simulink model "CVSDSpring2020Development"  (R2019a)
settings: Solver=FixedStepAuto  StartTime=0.0  StopTime=1.0  RelTol=1e-3
undefined symbols (not defined in the file or in its folder): DiscIntNeverNeededParam
settings Model: Creator=Dave  LastModifiedBy=Dave
settings DataIOCC: ReturnWorkspaceOutputs=off
settings DebuggingCC: ArithmeticOperatorsInVariantConditions=warning
settings SFSimCC: SimUseLocalCustomCode=off
settings RTWCC: RTWUseLocalCustomCode=off
settings CodeAppCC: StateflowObjectComments=on

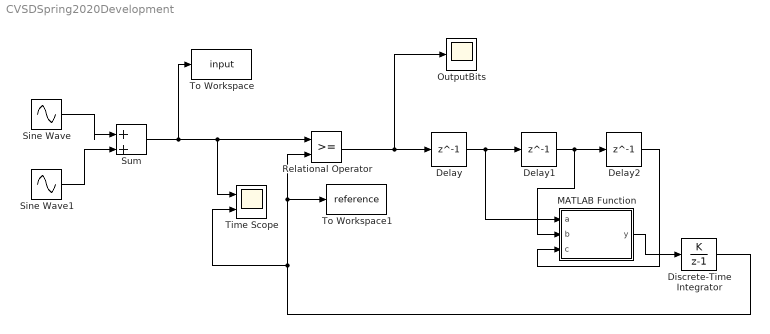
== system CVSDSpring2020Development ==
  Delay : Delay  DelayLength=1  InitialCondition=0
  Delay1 : Delay  DelayLength=1  InitialCondition=0
  Delay2 : Delay  DelayLength=1  InitialCondition=0
  Discrete-Time Integrator : DiscreteIntegrator  IntegratorMethod=Accumulation: Forward Euler  gainval=1  SampleTime=-1  ICPrevOutput=DiscIntNeverNeededParam  ICPrevScaledInput=DiscIntNeverNeededParam
  MATLAB Function : MATLAB Function  TreatAsAtomicUnit=on
  OutputBits : Scope
  Relational Operator : RelationalOperator  OutDataTypeStr=boolean  RndMeth=Simplest
  Sine Wave : Sin  Frequency=2*pi*1000  SampleTime=1/48e3
  Sine Wave1 : Sin  Frequency=2*pi*4000  SampleTime=1/48e3
  Sum : Sum  Inputs=|++
  Time Scope : Scope  NumInputPorts=2
  To Workspace : ToWorkspace  VariableName=input  SampleTime=-1
  To Workspace1 : ToWorkspace  VariableName=reference  SampleTime=-1
  wires:
  Relational Operator/1 -> Delay/1, OutputBits/1
  Sum/1 -> To Workspace/1, Time Scope/1, Relational Operator/1
  Sine Wave/1 -> Sum/1
  Sine Wave1/1 -> Sum/2
  Delay/1 -> MATLAB Function/1(a), Delay1/1
  Delay1/1 -> MATLAB Function/2(b), Delay2/1
  MATLAB Function/1(y) -> Discrete-Time Integrator/1
  Discrete-Time Integrator/1 -> Time Scope/2, To Workspace1/1, Relational Operator/2
  Delay2/1 -> MATLAB Function/3(c)

== matlab function CVSDSpring2020Development/MATLAB Function ==
  data: a input; y output; b input; c input
function y = fcn(a, b, c)

if a == 1
    y = 0.2;
else
    y = -0.2;
end

% run of 3 logic, boost pulse amplitude by 2x
if (a + b + c) == 3
    y = y * 2;
end
if (a + b + c) == 0
    y = y * 2;
end
